simulink model "power_mosfet_device"  (R2025b)
settings: Solver=ode23tb  StartTime=0.0  StopTime=simlength  MaxStep=tc  RelTol=1e-3
undefined symbols (not defined in the file or in its folder): mosfet
libraries: fl_lib x30, nesl_utility x15, simulink x2, advanced_mosfet_lib x1, basic_mosfet_lib x1
settings Model: SimulationMode=accelerator  Creator=dbagn  LastModifiedBy=dbagn

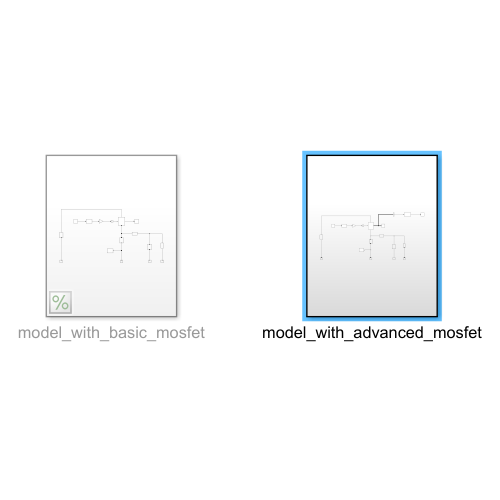
[thumbnail: Simulink's stored preview of the top-level diagram]
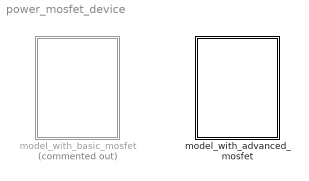
== system power_mosfet_device ==
  model_with_advanced_mosfet : Subsystem
  model_with_basic_mosfet : Subsystem  Commented=on

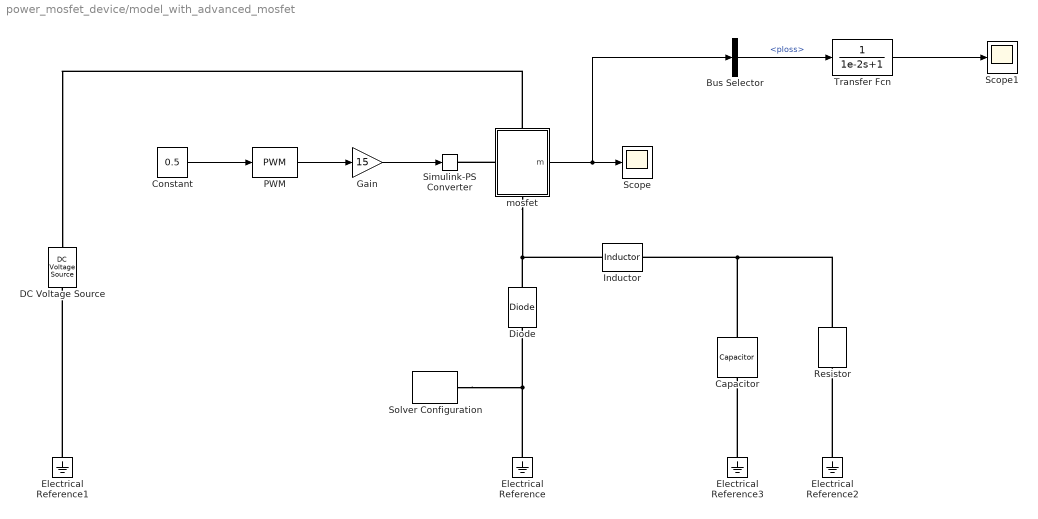
== system power_mosfet_device/model_with_advanced_mosfet ==
  Bus Selector : BusSelector  OutputSignals=basic_mosfet.ploss
  Capacitor : fl_lib/Electrical/Electrical Elements/Capacitor  c=200e-6 F  r=1e-6 Ohm  g=0 1/Ohm  i_specify=off  i_priority=None  i=0 A  i_nominal_specify=off  i_nominal_value=1  i_nominal_unit=A  v_specify=off  v_priority=None  v=0 V  v_nominal_specify=off  v_nominal_value=1  v_nominal_unit=V  vc_specify=off  vc_priority=High  vc=0 V  vc_nominal_specify=off  vc_nominal_value=1  vc_nominal_unit=V
  Constant : Constant  Value=0.5
  DC Voltage Source : fl_lib/Electrical/Electrical Sources/DC Voltage Source  v0=600 V
  Diode : fl_lib/Electrical/Electrical Elements/Diode  Vf=0.35 V  Ron=1e-3 Ohm  Goff=1e-8 1/Ohm  i_specify=off  i_priority=None  i=0 A  i_nominal_specify=off  i_nominal_value=1  i_nominal_unit=A  v_specify=off  v_priority=None  v=0 V  v_nominal_specify=off  v_nominal_value=1  v_nominal_unit=V
  Electrical Reference{,1..3} (4 alike) : fl_lib/Electrical/Electrical Elements/Electrical Reference
  Gain : Gain  Gain=15
  Inductor : fl_lib/Electrical/Electrical Elements/Inductor  l=400e-6 H  r=200e-3 Ohm  g=1e-9 1/Ohm  i_specify=off  i_priority=None  i=0 A  i_nominal_specify=off  i_nominal_value=1  i_nominal_unit=A  v_specify=off  v_priority=None  v=0 V  v_nominal_specify=off  v_nominal_value=1  v_nominal_unit=V  i_L_specify=off  i_L_priority=High  i_L=0 A  i_L_nominal_specify=off  i_L_nominal_value=1  i_L_nominal_unit=A
  PWM : simulink/Discontinuities/PWM  DisableCoverage=on  Period=1/10e3  InitialDelay=0  DisallowZeroDutyCycle=off  RunAtFixedTimeIntervals=off  SampleTime=0.1
  Resistor : fl_lib/Electrical/Electrical Elements/Resistor  R=300/200 Ohm  i_specify=off  i_priority=None  i=0 A  i_nominal_specify=off  i_nominal_value=1  i_nominal_unit=A  v_specify=off  v_priority=None  v=0 V  v_nominal_specify=off  v_nominal_value=1  v_nominal_unit=V
  Scope : Scope
      settings: SampleTime=tc  ActiveDisplayYMinimum=-140.53489713541944  ActiveDisplayYMaximum=839.36880778168631
  Scope1 : Scope
      settings: ActiveDisplayYMinimum=-40.413905236880076  ActiveDisplayYMaximum=363.72514713192072
  Simulink-PS Converter : nesl_utility/Simulink-PS Converter  PhysicalDomain=network_engine_domain  SubClassName=ps_input  LeftPortType=input  RightPortType=output  PseudoPeriodic=off  Frequencies=[]  NoiseDistribution=none  NoiseParameters=[]  Unit=1  AffineConversion=off  FilteringAndDerivatives=provide  SimscapeFilterOrder=1  InputFilterTimeConstant=0.001  UdotUserProvided=0
  Solver Configuration : nesl_utility/Solver Configuration  PhysicalDomain=network_engine_domain  SubClassName=solver  LeftPortType=input  RightPortType=generic  Tones=[]  Harmonics=[]  SimulateNoise=off  Profile=off  UseLocalSampling=off  EnableSwitchedLinearOptims=on  FrequencyDomain=off  UseCCode=off  RelTol=0.001  AbsTol=0.001  MinStep=1e-09  ToWorkspace=off  RevertToSquareIcSolve=off  NumHomotopyIterations=100  PhasorMode=off  PhasorModeNumHarmonics=1  ConsistencySolver=NEWTON_XTOL_AFTER_FTOL  IndexReductionMethod=DerivativeReplacement  DoDC=on  ResidualTolerance=1e-09  ConsistencyTolSource=GLOBAL  ConsistencyAbsTol=0.001  ConsistencyRelTol=0.001  ConsistencyTolFactor=0.001  UseLocalSolver=on  LocalSolverChoice=NE_BACKWARD_EULER_ADVANCER  ResolveIndetEquations=on  FunctionEvalNumThread=1  LocalSolverSampleTime=tc  DoFixedCost=on  MaxNonlinIter=3  MaxModeIter=2  ComputeImpulses=off  ImpulseIterations=2  LinearAlgebra=auto  LinearAlgebraNumThread=0  EquationFormulation=NE_TIME_EF  DelaysMemoryBudget=1024  AutomaticFiltering=on  FilteringTimeConstant=0.001  PartitionStorageMethod=AS_NEEDED  PartitionMemoryBudget=1024  PartitionMethod=ROBUST  MultibodyUseLocalSolver=off  MultibodyLocalSolverChoice=ODE1  MultibodyLocalSolverSampleTime=0.001
  Transfer Fcn : TransferFcn  Denominator=[1e-2 1]
  mosfet : Subsystem  mask{Rds_on=mosfet.inv.Rds_on, Vth=mosfet.inv.Vth, Csnubber=mosfet.inv.Csnubber, Rsnubber=mosfet.inv.Rsnubber, Lstray=mosfet.inv.Lstray_module/2, Vdon_diode=mosfet.inv.Vdon_diode, Rdon_diode=mosfet.inv.Rdon_diode, g_fs=150, Ciss=mosfet.inv.Ciss, Coss=mosfet.inv.Coss, Crss=mosfet.inv.Crss, Rgate_internal=1, Rgate_external=1}
      mask prompts: Rds_on "Rds_on (Ohm)"; Vth "Vth (V)"; Csnubber "Csnubber (F)"; Rsnubber "Rsnubber (Ohm)"; Lstray "Lstray (H)"; Vdon_diode "Vdon_diode (V)"; Rdon_diode "Rdon_diode (Ohm)"; g_fs "g_fs (A/V)"; Ciss "Ciss (F)"; Coss "Coss (F)"; Crss "Crss (F)"; Rgate_internal "Rgate internal (Ohm)"; Rgate_external "Rgate external (Ohm)"
      settings: PortSchema="{\"entries\":[{\"content\":{\"sides\":[{\"content\":{\"connectorIds\":[\"LConn1\"]},\"type\":\"ConnectorPlacement.EquallySpacedRectSide\",\"uuid\":\"325dc963-858c-47f0-8995-f323ab4d9c46\"},{\"content\":{\"connectorIds\":[\"Out1\"],\"side\":\"RIGHT\"},\"type\":\"ConnectorPlacement.EquallySpacedRectSide\",\"uuid\":\"e9e66084-ecb2-40fb-9a1e-77677e0cc1df\"},{\"content\":{\"connectorIds\":[\"LConn2\"],\"side\":\"TOP\"},\"type\":\"ConnectorPlacement.EquallySpacedRectSide\",\"uuid\":\"9480d797-f2f6-459b-bb7c-d63861b57fde\"},{\"content\":{\"connectorIds\":[\"RConn1\"],\"side\":\"BOTTOM\"},\"type\":\"ConnectorPlacement.EquallySpacedRectSide\",\"uuid\":\"b13176d9-73b9-4822-9a0d-ec75065272bc\"}]},\"type\":\"ConnectorPlacement.EquallySpacedConnector\",\"uuid\":\"5e4a07d9-f5e8-4613-9049-5a866b5d2453\"}],\"packageUris\":[\"http://schema.mathworks.com/mf0/Connector/R2020b\"],\"version\":\"1.0\"}"
  wires:
  Gain/1 -> Simulink-PS Converter/1
  mosfet/1(m) -> Bus Selector/1, Scope/1
  Constant/1 -> PWM/1
  PWM/1 -> Gain/1
  Bus Selector/1 -> Transfer Fcn/1  "<ploss>"
  Transfer Fcn/1 -> Scope1/1
  connections:
  Electrical Reference1/LConn1 -- DC Voltage Source/RConn1
  mosfet/LConn1 -- Simulink-PS Converter/RConn1
  mosfet/LConn2 -- Diode/RConn1 -- Inductor/LConn1
  Capacitor/LConn1 -- Resistor/LConn1 -- Inductor/RConn1
  Electrical Reference2/LConn1 -- Resistor/RConn1
  Electrical Reference3/LConn1 -- Capacitor/RConn1
  Solver Configuration/RConn1 -- Electrical Reference/LConn1 -- Diode/LConn1
  mosfet/RConn1 -- DC Voltage Source/LConn1

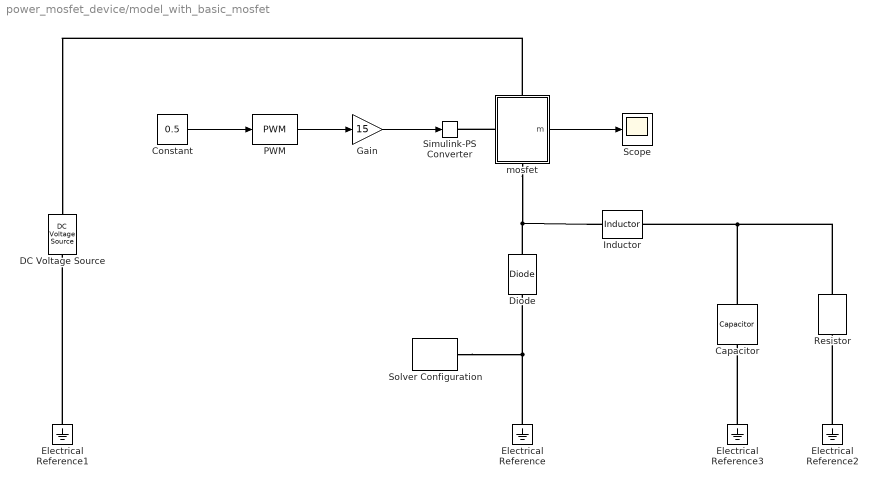
== system power_mosfet_device/model_with_basic_mosfet ==
  Capacitor : fl_lib/Electrical/Electrical Elements/Capacitor  c=200e-6 F  r=1e-6 Ohm  g=0 1/Ohm  i_specify=off  i_priority=None  i=0 A  i_nominal_specify=off  i_nominal_value=1  i_nominal_unit=A  v_specify=off  v_priority=None  v=0 V  v_nominal_specify=off  v_nominal_value=1  v_nominal_unit=V  vc_specify=off  vc_priority=High  vc=0 V  vc_nominal_specify=off  vc_nominal_value=1  vc_nominal_unit=V
  Constant : Constant  Value=0.5
  DC Voltage Source : fl_lib/Electrical/Electrical Sources/DC Voltage Source  v0=600 V
  Diode : fl_lib/Electrical/Electrical Elements/Diode  Vf=0.35 V  Ron=1e-3 Ohm  Goff=1e-8 1/Ohm  i_specify=off  i_priority=None  i=0 A  i_nominal_specify=off  i_nominal_value=1  i_nominal_unit=A  v_specify=off  v_priority=None  v=0 V  v_nominal_specify=off  v_nominal_value=1  v_nominal_unit=V
  Electrical Reference{,1..3} (4 alike) : fl_lib/Electrical/Electrical Elements/Electrical Reference
  Gain : Gain  Gain=15
  Inductor : fl_lib/Electrical/Electrical Elements/Inductor  l=400e-6 H  r=200e-3 Ohm  g=1e-9 1/Ohm  i_specify=off  i_priority=None  i=0 A  i_nominal_specify=off  i_nominal_value=1  i_nominal_unit=A  v_specify=off  v_priority=None  v=0 V  v_nominal_specify=off  v_nominal_value=1  v_nominal_unit=V  i_L_specify=off  i_L_priority=High  i_L=0 A  i_L_nominal_specify=off  i_L_nominal_value=1  i_L_nominal_unit=A
  PWM : simulink/Discontinuities/PWM  DisableCoverage=on  Period=1/10e3  InitialDelay=0  DisallowZeroDutyCycle=off  RunAtFixedTimeIntervals=off  SampleTime=0.1
  Resistor : fl_lib/Electrical/Electrical Elements/Resistor  R=300/200 Ohm  i_specify=off  i_priority=None  i=0 A  i_nominal_specify=off  i_nominal_value=1  i_nominal_unit=A  v_specify=off  v_priority=None  v=0 V  v_nominal_specify=off  v_nominal_value=1  v_nominal_unit=V
  Scope : Scope
      settings: SampleTime=tc  ActiveDisplayYMinimum=-140.53489713541944  ActiveDisplayYMaximum=839.36880778168631
  Simulink-PS Converter : nesl_utility/Simulink-PS Converter  PhysicalDomain=network_engine_domain  SubClassName=ps_input  LeftPortType=input  RightPortType=output  PseudoPeriodic=off  Frequencies=[]  NoiseDistribution=none  NoiseParameters=[]  Unit=1  AffineConversion=off  FilteringAndDerivatives=provide  SimscapeFilterOrder=1  InputFilterTimeConstant=0.001  UdotUserProvided=0
  Solver Configuration : nesl_utility/Solver Configuration  PhysicalDomain=network_engine_domain  SubClassName=solver  LeftPortType=input  RightPortType=generic  Tones=[]  Harmonics=[]  SimulateNoise=off  Profile=off  UseLocalSampling=off  EnableSwitchedLinearOptims=on  FrequencyDomain=off  UseCCode=off  RelTol=0.001  AbsTol=0.001  MinStep=1e-09  ToWorkspace=off  RevertToSquareIcSolve=off  NumHomotopyIterations=100  PhasorMode=off  PhasorModeNumHarmonics=1  ConsistencySolver=NEWTON_XTOL_AFTER_FTOL  IndexReductionMethod=DerivativeReplacement  DoDC=on  ResidualTolerance=1e-09  ConsistencyTolSource=GLOBAL  ConsistencyAbsTol=0.001  ConsistencyRelTol=0.001  ConsistencyTolFactor=0.001  UseLocalSolver=on  LocalSolverChoice=NE_BACKWARD_EULER_ADVANCER  ResolveIndetEquations=on  FunctionEvalNumThread=1  LocalSolverSampleTime=tc  DoFixedCost=on  MaxNonlinIter=3  MaxModeIter=2  ComputeImpulses=off  ImpulseIterations=2  LinearAlgebra=auto  LinearAlgebraNumThread=0  EquationFormulation=NE_TIME_EF  DelaysMemoryBudget=1024  AutomaticFiltering=on  FilteringTimeConstant=0.001  PartitionStorageMethod=AS_NEEDED  PartitionMemoryBudget=1024  PartitionMethod=ROBUST  MultibodyUseLocalSolver=off  MultibodyLocalSolverChoice=ODE1  MultibodyLocalSolverSampleTime=0.001
  mosfet : Subsystem  mask{Rds_on=mosfet.inv.Rds_on, Vth=mosfet.inv.Vth, Csnubber=mosfet.inv.Csnubber, Rsnubber=mosfet.inv.Rsnubber, Lstray=mosfet.inv.Lstray_module/2, Vdon_diode=mosfet.inv.Vdon_diode, Rdon_diode=mosfet.inv.Rdon_diode, g_fs=150}
      mask prompts: Rds_on "Rds_on (Ohm)"; Vth "Vth (V)"; Csnubber "Csnubber (F)"; Rsnubber "Rsnubber (Ohm)"; Lstray "Lstray (H)"; Vdon_diode "Vdon_diode (V)"; Rdon_diode "Rdon_diode (Ohm)"; g_fs "g_fs (A/V)"
      settings: PortSchema="{\"entries\":[{\"content\":{\"sides\":[{\"content\":{\"connectorIds\":[\"LConn1\"]},\"type\":\"ConnectorPlacement.EquallySpacedRectSide\",\"uuid\":\"325dc963-858c-47f0-8995-f323ab4d9c46\"},{\"content\":{\"connectorIds\":[\"Out1\"],\"side\":\"RIGHT\"},\"type\":\"ConnectorPlacement.EquallySpacedRectSide\",\"uuid\":\"e9e66084-ecb2-40fb-9a1e-77677e0cc1df\"},{\"content\":{\"connectorIds\":[\"LConn2\"],\"side\":\"TOP\"},\"type\":\"ConnectorPlacement.EquallySpacedRectSide\",\"uuid\":\"9480d797-f2f6-459b-bb7c-d63861b57fde\"},{\"content\":{\"connectorIds\":[\"RConn1\"],\"side\":\"BOTTOM\"},\"type\":\"ConnectorPlacement.EquallySpacedRectSide\",\"uuid\":\"b13176d9-73b9-4822-9a0d-ec75065272bc\"}]},\"type\":\"ConnectorPlacement.EquallySpacedConnector\",\"uuid\":\"5e4a07d9-f5e8-4613-9049-5a866b5d2453\"}],\"packageUris\":[\"http://schema.mathworks.com/mf0/Connector/R2020b\"],\"version\":\"1.0\"}"
  wires:
  PWM/1 -> Gain/1
  Constant/1 -> PWM/1
  mosfet/1(m) -> Scope/1
  Gain/1 -> Simulink-PS Converter/1
  connections:
  mosfet/RConn1 -- DC Voltage Source/LConn1
  Electrical Reference/LConn1 -- Solver Configuration/RConn1 -- Diode/LConn1
  Electrical Reference3/LConn1 -- Capacitor/RConn1
  Electrical Reference2/LConn1 -- Resistor/RConn1
  Resistor/LConn1 -- Capacitor/LConn1 -- Inductor/RConn1
  Diode/RConn1 -- mosfet/LConn2 -- Inductor/LConn1
  mosfet/LConn1 -- Simulink-PS Converter/RConn1
  Electrical Reference1/LConn1 -- DC Voltage Source/RConn1

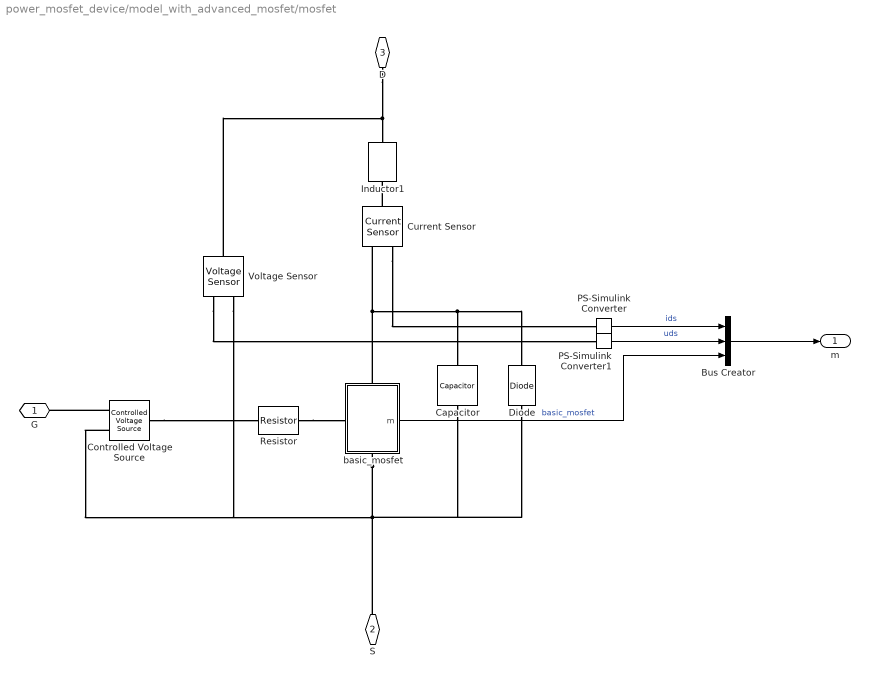
== system power_mosfet_device/model_with_advanced_mosfet/mosfet ==
  Bus Creator : BusCreator  Inputs=3
  Capacitor : fl_lib/Electrical/Electrical Elements/Capacitor  c=Csnubber F  r=Rsnubber Ohm  g=0 1/Ohm  i_specify=off  i_priority=None  i=0 A  i_nominal_specify=off  i_nominal_value=1  i_nominal_unit=A  v_specify=off  v_priority=None  v=0 V  v_nominal_specify=off  v_nominal_value=1  v_nominal_unit=V  vc_specify=off  vc_priority=High  vc=0 V  vc_nominal_specify=off  vc_nominal_value=1  vc_nominal_unit=V
  Controlled Voltage Source : fl_lib/Electrical/Electrical Sources/Controlled Voltage Source
  Current Sensor : fl_lib/Electrical/Electrical Sensors/Current Sensor
  Diode : fl_lib/Electrical/Electrical Elements/Diode  Vf=Vdon_diode V  Ron=Rdon_diode Ohm  Goff=1e-8 1/Ohm  i_specify=off  i_priority=None  i=0 A  i_nominal_specify=off  i_nominal_value=1  i_nominal_unit=A  v_specify=off  v_priority=None  v=0 V  v_nominal_specify=off  v_nominal_value=1  v_nominal_unit=V
  Inductor1 : fl_lib/Electrical/Electrical Elements/Inductor  l=Lstray H  r=0 Ohm  g=1e-9 1/Ohm  i_specify=off  i_priority=None  i=0 A  i_nominal_specify=off  i_nominal_value=1  i_nominal_unit=A  v_specify=off  v_priority=None  v=0 V  v_nominal_specify=off  v_nominal_value=1  v_nominal_unit=V  i_L_specify=off  i_L_priority=High  i_L=0 A  i_L_nominal_specify=off  i_L_nominal_value=1  i_L_nominal_unit=A
  PS-Simulink Converter : nesl_utility/PS-Simulink Converter  PhysicalDomain=network_engine_domain  SubClassName=ps_output  LeftPortType=input  RightPortType=output  PseudoPeriodic=off  Frequencies=[]  VectorFormat=1-D array  Unit=A  AffineConversion=off
  PS-Simulink Converter1 : nesl_utility/PS-Simulink Converter  PhysicalDomain=network_engine_domain  SubClassName=ps_output  LeftPortType=input  RightPortType=output  PseudoPeriodic=off  Frequencies=[]  VectorFormat=1-D array  Unit=V  AffineConversion=off
  Resistor : fl_lib/Electrical/Electrical Elements/Resistor  R=Rgate_external Ohm  i_specify=off  i_priority=None  i=0 A  i_nominal_specify=off  i_nominal_value=1  i_nominal_unit=A  v_specify=off  v_priority=None  v=0 V  v_nominal_specify=off  v_nominal_value=1  v_nominal_unit=V
  Voltage Sensor : fl_lib/Electrical/Electrical Sensors/Voltage Sensor
  basic_mosfet : Subsystem  mask{Vth=Vth, Rds_on=Rds_on, g_fs=g_fs, Ciss=Ciss, Crss=Crss, Coss=Coss, Rgate=Rgate_internal}
      mask prompts: Vth "Vth (V)"; Rds_on "Rds_on (Ohm)"; g_fs "g_fs (A/V)"; Ciss "Ciss (F)"; Crss "Crss (F)"; Coss "Coss (F)"; Rgate "Rgate internal (Ohm)"
      settings: PortSchema="{\"entries\":[{\"content\":{\"sides\":[{\"content\":{\"connectorIds\":[\"LConn1\"]},\"type\":\"ConnectorPlacement.EquallySpacedRectSide\",\"uuid\":\"325dc963-858c-47f0-8995-f323ab4d9c46\"},{\"content\":{\"connectorIds\":[\"Out1\"],\"side\":\"RIGHT\"},\"type\":\"ConnectorPlacement.EquallySpacedRectSide\",\"uuid\":\"e9e66084-ecb2-40fb-9a1e-77677e0cc1df\"},{\"content\":{\"connectorIds\":[\"LConn2\"],\"side\":\"TOP\"},\"type\":\"ConnectorPlacement.EquallySpacedRectSide\",\"uuid\":\"9480d797-f2f6-459b-bb7c-d63861b57fde\"},{\"content\":{\"connectorIds\":[\"RConn1\"],\"side\":\"BOTTOM\"},\"type\":\"ConnectorPlacement.EquallySpacedRectSide\",\"uuid\":\"bd6f7c3f-e73f-43a3-8bfd-bc4aa1f2c71d\"}]},\"type\":\"ConnectorPlacement.EquallySpacedConnector\",\"uuid\":\"5e4a07d9-f5e8-4613-9049-5a866b5d2453\"}],\"packageUris\":[\"http://schema.mathworks.com/mf0/Connector/R2020b\"],\"version\":\"1.0\"}"
  G : PMIOPort  Side=Left
  S : PMIOPort  Port=2  Side=Left
  D : PMIOPort  Port=3  Side=Right
  m : Outport
  wires:
  basic_mosfet/1(m) -> Bus Creator/3  "basic_mosfet"
  Bus Creator/1 -> m/1
  PS-Simulink Converter/1 -> Bus Creator/1  "ids"
  PS-Simulink Converter1/1 -> Bus Creator/2  "uds"
  connections:
  Current Sensor/LConn1 -- Inductor1/LConn1
  Voltage Sensor/RConn1 -- PS-Simulink Converter1/LConn1
  Voltage Sensor/LConn1 -- Inductor1/RConn1 -- D/RConn1
  basic_mosfet/LConn2 -- Diode/RConn1 -- Capacitor/LConn1 -- Current Sensor/RConn2
  Current Sensor/RConn1 -- PS-Simulink Converter/LConn1
  basic_mosfet/RConn1 -- Controlled Voltage Source/RConn2 -- Voltage Sensor/RConn2 -- S/RConn1 -- Capacitor/RConn1 -- Diode/LConn1
  Controlled Voltage Source/RConn1 -- G/RConn1
  Controlled Voltage Source/LConn1 -- Resistor/LConn1
  Resistor/RConn1 -- basic_mosfet/LConn1

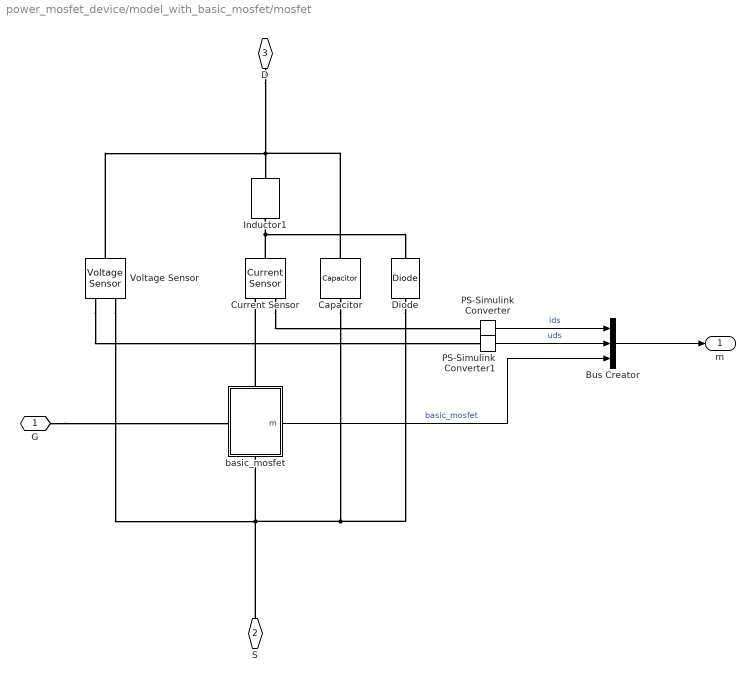
== system power_mosfet_device/model_with_basic_mosfet/mosfet ==
  Bus Creator : BusCreator  Inputs=3
  Capacitor : fl_lib/Electrical/Electrical Elements/Capacitor  c=Csnubber F  r=Rsnubber Ohm  g=0 1/Ohm  i_specify=off  i_priority=None  i=0 A  i_nominal_specify=off  i_nominal_value=1  i_nominal_unit=A  v_specify=off  v_priority=None  v=0 V  v_nominal_specify=off  v_nominal_value=1  v_nominal_unit=V  vc_specify=off  vc_priority=High  vc=0 V  vc_nominal_specify=off  vc_nominal_value=1  vc_nominal_unit=V
  Current Sensor : fl_lib/Electrical/Electrical Sensors/Current Sensor
  Diode : fl_lib/Electrical/Electrical Elements/Diode  Vf=Vdon_diode V  Ron=Rdon_diode Ohm  Goff=1e-8 1/Ohm  i_specify=off  i_priority=None  i=0 A  i_nominal_specify=off  i_nominal_value=1  i_nominal_unit=A  v_specify=off  v_priority=None  v=0 V  v_nominal_specify=off  v_nominal_value=1  v_nominal_unit=V
  Inductor1 : fl_lib/Electrical/Electrical Elements/Inductor  l=Lstray H  r=0 Ohm  g=1e-9 1/Ohm  i_specify=off  i_priority=None  i=0 A  i_nominal_specify=off  i_nominal_value=1  i_nominal_unit=A  v_specify=off  v_priority=None  v=0 V  v_nominal_specify=off  v_nominal_value=1  v_nominal_unit=V  i_L_specify=off  i_L_priority=High  i_L=0 A  i_L_nominal_specify=off  i_L_nominal_value=1  i_L_nominal_unit=A
  PS-Simulink Converter : nesl_utility/PS-Simulink Converter  PhysicalDomain=network_engine_domain  SubClassName=ps_output  LeftPortType=input  RightPortType=output  PseudoPeriodic=off  Frequencies=[]  VectorFormat=1-D array  Unit=A  AffineConversion=off
  PS-Simulink Converter1 : nesl_utility/PS-Simulink Converter  PhysicalDomain=network_engine_domain  SubClassName=ps_output  LeftPortType=input  RightPortType=output  PseudoPeriodic=off  Frequencies=[]  VectorFormat=1-D array  Unit=V  AffineConversion=off
  Voltage Sensor : fl_lib/Electrical/Electrical Sensors/Voltage Sensor
  basic_mosfet : Subsystem  mask{Vth=Vth, Rds_on=Rds_on, g_fs=g_fs}
      mask prompts: Vth "Vth (V)"; Rds_on "Rds_on (Ohm)"; g_fs "g_fs (A/V)"
      settings: PortSchema="{\"entries\":[{\"content\":{\"sides\":[{\"content\":{\"connectorIds\":[\"LConn1\"]},\"type\":\"ConnectorPlacement.EquallySpacedRectSide\",\"uuid\":\"325dc963-858c-47f0-8995-f323ab4d9c46\"},{\"content\":{\"connectorIds\":[\"Out1\"],\"side\":\"RIGHT\"},\"type\":\"ConnectorPlacement.EquallySpacedRectSide\",\"uuid\":\"e9e66084-ecb2-40fb-9a1e-77677e0cc1df\"},{\"content\":{\"connectorIds\":[\"LConn2\"],\"side\":\"TOP\"},\"type\":\"ConnectorPlacement.EquallySpacedRectSide\",\"uuid\":\"9480d797-f2f6-459b-bb7c-d63861b57fde\"},{\"content\":{\"connectorIds\":[\"RConn1\"],\"side\":\"BOTTOM\"},\"type\":\"ConnectorPlacement.EquallySpacedRectSide\",\"uuid\":\"bd6f7c3f-e73f-43a3-8bfd-bc4aa1f2c71d\"}]},\"type\":\"ConnectorPlacement.EquallySpacedConnector\",\"uuid\":\"5e4a07d9-f5e8-4613-9049-5a866b5d2453\"}],\"packageUris\":[\"http://schema.mathworks.com/mf0/Connector/R2020b\"],\"version\":\"1.0\"}"
  G : PMIOPort  Side=Left
  S : PMIOPort  Port=2  Side=Left
  D : PMIOPort  Port=3  Side=Right
  m : Outport
  wires:
  PS-Simulink Converter1/1 -> Bus Creator/2  "uds"
  PS-Simulink Converter/1 -> Bus Creator/1  "ids"
  Bus Creator/1 -> m/1
  basic_mosfet/1(m) -> Bus Creator/3  "basic_mosfet"
  connections:
  Diode/LConn1 -- Capacitor/RConn1 -- Voltage Sensor/RConn2 -- basic_mosfet/RConn1 -- S/RConn1
  Current Sensor/RConn1 -- PS-Simulink Converter/LConn1
  basic_mosfet/LConn2 -- Current Sensor/RConn2
  G/RConn1 -- basic_mosfet/LConn1
  Capacitor/LConn1 -- D/RConn1 -- Voltage Sensor/LConn1 -- Inductor1/RConn1
  Voltage Sensor/RConn1 -- PS-Simulink Converter1/LConn1
  Current Sensor/LConn1 -- Diode/RConn1 -- Inductor1/LConn1

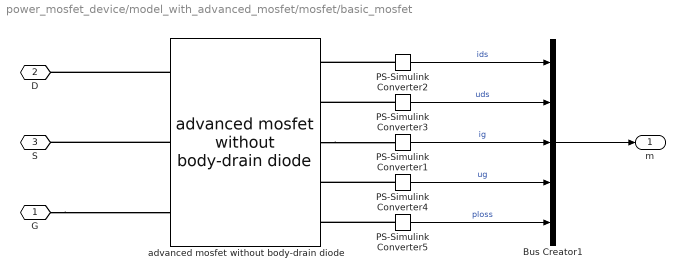
== system power_mosfet_device/model_with_advanced_mosfet/mosfet/basic_mosfet ==
  Bus Creator1 : BusCreator  Inputs=5
  PS-Simulink Converter1 : nesl_utility/PS-Simulink Converter  PhysicalDomain=network_engine_domain  SubClassName=ps_output  LeftPortType=input  RightPortType=output  PseudoPeriodic=off  Frequencies=[]  VectorFormat=1-D array  Unit=A  AffineConversion=off
  PS-Simulink Converter2 : nesl_utility/PS-Simulink Converter  PhysicalDomain=network_engine_domain  SubClassName=ps_output  LeftPortType=input  RightPortType=output  PseudoPeriodic=off  Frequencies=[]  VectorFormat=1-D array  Unit=A  AffineConversion=off
  PS-Simulink Converter3 : nesl_utility/PS-Simulink Converter  PhysicalDomain=network_engine_domain  SubClassName=ps_output  LeftPortType=input  RightPortType=output  PseudoPeriodic=off  Frequencies=[]  VectorFormat=1-D array  Unit=V  AffineConversion=off
  PS-Simulink Converter4 : nesl_utility/PS-Simulink Converter  PhysicalDomain=network_engine_domain  SubClassName=ps_output  LeftPortType=input  RightPortType=output  PseudoPeriodic=off  Frequencies=[]  VectorFormat=1-D array  Unit=V  AffineConversion=off
  PS-Simulink Converter5 : nesl_utility/PS-Simulink Converter  PhysicalDomain=network_engine_domain  SubClassName=ps_output  LeftPortType=input  RightPortType=output  PseudoPeriodic=off  Frequencies=[]  VectorFormat=1-D array  Unit=W  AffineConversion=off
  advanced mosfet without body-drain diode : advanced_mosfet_lib/advanced mosfet without body-drain diode  Vth=Vth V  g_fs=g_fs A/V  Rds_on=Rds_on Ohm  Cgs=Ciss F  Cgd=Crss F  Cds=Coss F  Rg=Rgate Ohm  ids_i_specify=off  ids_i_priority=None  ids_i=0 A  ids_i_nominal_specify=off  ids_i_nominal_value=1  ids_i_nominal_unit=A  ids_ii_specify=off  ids_ii_priority=None  ids_ii=0 A  ids_ii_nominal_specify=off  ids_ii_nominal_value=1  ids_ii_nominal_unit=A  idsi_specify=off  idsi_priority=High  idsi=0 A  idsi_nominal_specify=off  idsi_nominal_value=1  idsi_nominal_unit=A  icgs_specify=off  icgs_priority=None  icgs=0 A  icgs_nominal_specify=off  icgs_nominal_value=1  icgs_nominal_unit=A  icgd_specify=off  icgd_priority=None  icgd=0 A  icgd_nominal_specify=off  icgd_nominal_value=1  icgd_nominal_unit=A  icds_specify=off  icds_priority=None  icds=0 A  icds_nominal_specify=off  icds_nominal_value=1  icds_nominal_unit=A  ugs_specify=off  ugs_priority=None  ugs=0 V  ugs_nominal_specify=off  ugs_nominal_value=1  ugs_nominal_unit=V  uds_specify=off  uds_priority=None  uds=0 V  uds_nominal_specify=off  uds_nominal_value=1  uds_nominal_unit=V  ucgs_specify=off  ucgs_priority=None  ucgs=0 V  ucgs_nominal_specify=off  ucgs_nominal_value=1  ucgs_nominal_unit=V  ucgd_specify=off  ucgd_priority=None  ucgd=0 V  ucgd_nominal_specify=off  ucgd_nominal_value=1  ucgd_nominal_unit=V  udsi_specify=off  udsi_priority=None  udsi=0 V  udsi_nominal_specify=off  udsi_nominal_value=1  udsi_nominal_unit=V  igs_specify=off  igs_priority=High  igs=0 A  igs_nominal_specify=off  igs_nominal_value=1  igs_nominal_unit=A  idsi_active_specify=off  idsi_active_priority=None  idsi_active=0 A  idsi_active_nominal_specify=off  idsi_active_nominal_value=1  idsi_active_nominal_unit=A  idsi_on_specify=off  idsi_on_priority=None  idsi_on=0 A  idsi_on_nominal_specify=off  idsi_on_nominal_value=1  idsi_on_nominal_unit=A
      settings: InternalSimscapePortConfiguration="{\"Bottom\":[],\"Left\":[{\"id\":\"D\",\"label\":\"D\",\"type\":\"foundation.electrical.electrical\"},{\"id\":\"S\",\"label\":\"S\",\"type\":\"foundation.electrical.electrical\"},{\"id\":\"G\",\"label\":\"G\",\"type\":\"foundation.electrical.electrical\"}],\"Right\":[{\"id\":\"idsi_out\",\"label\":\"ids\",\"type\":\"output\"},{\"id\":\"udsi_out\",\"label\":\"uds\",\"type\":\"output\"},{\"id\":\"igs_out\",\"label\":\"igs\",\"type\":\"output\"},{\"id\":\"ugs_out\",\"label\":\"ugs\",\"type\":\"output\"},{\"id\":\"p_device\",\"label\":\"ploss\",\"type\":\"output\"}],\"Top\":[]}"
  G : PMIOPort  Side=Left
  D : PMIOPort  Port=2  Side=Left
  S : PMIOPort  Port=3  Side=Right
  m : Outport
  wires:
  Bus Creator1/1 -> m/1
  PS-Simulink Converter2/1 -> Bus Creator1/1  "ids"
  PS-Simulink Converter3/1 -> Bus Creator1/2  "uds"
  PS-Simulink Converter1/1 -> Bus Creator1/3  "ig"
  PS-Simulink Converter4/1 -> Bus Creator1/4  "ug"
  PS-Simulink Converter5/1 -> Bus Creator1/5  "ploss"
  connections:
  PS-Simulink Converter3/LConn1 -- advanced mosfet without body-drain diode/RConn2
  PS-Simulink Converter2/LConn1 -- advanced mosfet without body-drain diode/RConn1
  advanced mosfet without body-drain diode/LConn1 -- D/RConn1
  advanced mosfet without body-drain diode/LConn2 -- S/RConn1
  G/RConn1 -- advanced mosfet without body-drain diode/LConn3
  PS-Simulink Converter4/LConn1 -- advanced mosfet without body-drain diode/RConn4
  advanced mosfet without body-drain diode/RConn3 -- PS-Simulink Converter1/LConn1
  PS-Simulink Converter5/LConn1 -- advanced mosfet without body-drain diode/RConn5

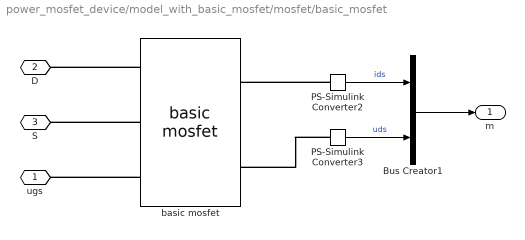
== system power_mosfet_device/model_with_basic_mosfet/mosfet/basic_mosfet ==
  Bus Creator1 : BusCreator  Inputs=2
  PS-Simulink Converter2 : nesl_utility/PS-Simulink Converter  PhysicalDomain=network_engine_domain  SubClassName=ps_output  LeftPortType=input  RightPortType=output  PseudoPeriodic=off  Frequencies=[]  VectorFormat=1-D array  Unit=A  AffineConversion=off
  PS-Simulink Converter3 : nesl_utility/PS-Simulink Converter  PhysicalDomain=network_engine_domain  SubClassName=ps_output  LeftPortType=input  RightPortType=output  PseudoPeriodic=off  Frequencies=[]  VectorFormat=1-D array  Unit=V  AffineConversion=off
  basic mosfet : basic_mosfet_lib/basic mosfet  Vth=Vth V  g_fs=g_fs A/V  Rds_on=Rds_on Ohm  ids_specify=off  ids_priority=High  ids=0 A  ids_nominal_specify=off  ids_nominal_value=1  ids_nominal_unit=A  uds_specify=off  uds_priority=None  uds=0 V  uds_nominal_specify=off  uds_nominal_value=1  uds_nominal_unit=V  ib_specify=off  ib_priority=None  ib=0 A  ib_nominal_specify=off  ib_nominal_value=1  ib_nominal_unit=A  ids_on_specify=off  ids_on_priority=None  ids_on=0 A  ids_on_nominal_specify=off  ids_on_nominal_value=1  ids_on_nominal_unit=A
      settings: InternalSimscapePortConfiguration="{\"Bottom\":[],\"Left\":[{\"id\":\"D\",\"label\":\"D\",\"type\":\"foundation.electrical.electrical\"},{\"id\":\"S\",\"label\":\"S\",\"type\":\"foundation.electrical.electrical\"},{\"id\":\"ugs\",\"label\":\"ugs\",\"type\":\"input\"}],\"Right\":[{\"id\":\"ids_out\",\"label\":\"ids\",\"type\":\"output\"},{\"id\":\"uds_out\",\"label\":\"uds\",\"type\":\"output\"}],\"Top\":[]}"
  ugs : PMIOPort  Side=Left
  D : PMIOPort  Port=2  Side=Left
  S : PMIOPort  Port=3  Side=Right
  m : Outport
  wires:
  PS-Simulink Converter3/1 -> Bus Creator1/2  "uds"
  PS-Simulink Converter2/1 -> Bus Creator1/1  "ids"
  Bus Creator1/1 -> m/1
  connections:
  basic mosfet/LConn3 -- ugs/RConn1
  basic mosfet/LConn1 -- D/RConn1
  PS-Simulink Converter2/LConn1 -- basic mosfet/RConn1
  basic mosfet/LConn2 -- S/RConn1
  PS-Simulink Converter3/LConn1 -- basic mosfet/RConn2
